simulink model "Raspi_LSTM"  (R2023a)
settings: Solver=FixedStepAuto  StartTime=0.0  StopTime=inf  RelTol=1e-3  EnableMultiTasking=on
InitFcn:
  | timespan=1.5;
  | sampling_subsample=3;
undefined symbols (not defined in the file or in its folder): plughw
libraries: dspvision x8, raspberrypiIOTlib x2, raspberrypiAVlib x1, dspsnks4 x1, deeplib x1, dspfeatures x1
settings Model: SimulationMode=external  ExtModeTrigDuration=2  Creator=tokamoto  LastModifiedBy=tokamoto
settings SolverCC: AlgebraicLoopSolver=TrustRegion  PositivePriorityOrder=on
settings DataIOCC: LimitDataPoints=on  DSMLogging=off  StreamToWks=off  ReturnWorkspaceOutputs=off
settings OptimizationCC: ZeroExternalMemoryAtStartup=off  ZeroInternalMemoryAtStartup=off  MaxStackSize=64
settings DebuggingCC: ParameterTunabilityLossMsg=error  UnconnectedInputMsg=warning  UnconnectedOutputMsg=warning  UnconnectedLineMsg=warning  ArithmeticOperatorsInVariantConditions=warning
settings HardwareCC: ProdBitPerPointer=32  ProdBitPerSizeT=32  ProdBitPerPtrDiffT=32  ProdLargestAtomicInteger=Long  ProdLargestAtomicFloat=Double  ProdWordSize=32  ProdLongLongMode=on  ProdHWDeviceType=ARM Compatible->ARM Cortex
settings ModelReferenceCC: EnableRefExpFcnMdlSchedulingChecks=on
settings SFSimCC: SimUseLocalCustomCode=off  CustomCodeUndefinedFunction=UseInterfaceOnly
settings RTWCC: Description=Embedded Coder  SystemTargetFile=ert.tlc  HardwareBoard=Raspberry Pi  TLCOptions="-aInlineSetEventsForThisBaseRateFcn=TLC_FALSE -aSuppressMultiTaskScheduler=TLC_FALSE  -aRateBasedStepFcn=0"  TemplateMakefile=ert_default_tmf  GenerateReport=on  RTWUseLocalCustomCode=off  Toolchain=GNU GCC Embedded Linux  BuildConfiguration=Faster Runs  LaunchReport=on  GenerateCodeMetricsReport=on
settings CodeAppCC: ForceParamTrailComments=on  OperatorAnnotations=on  StateflowObjectComments=on  MATLABSourceComments=on
settings ERTTargetCC: CodeReplacementLibrary=GCC ARM Cortex-A  ERTCustomFileBanners=off  SupportComplex=off  SupportNonInlinedSFcns=on  RemoveResetFunc=off  SupportVariableSizeSignals=on  ModelStepFunctionPrototypeControlCompliant=off  ExtModeTransport=2  ExtModeStaticAlloc=on  ExtModeMexFile=ext_xcp  ExtModeIntrfLevel=Level2 - Open  RootIOFormat=Structure reference

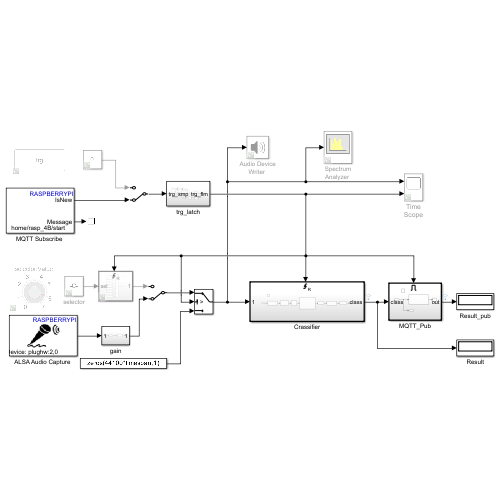
[thumbnail: Simulink's stored preview of the top-level diagram]
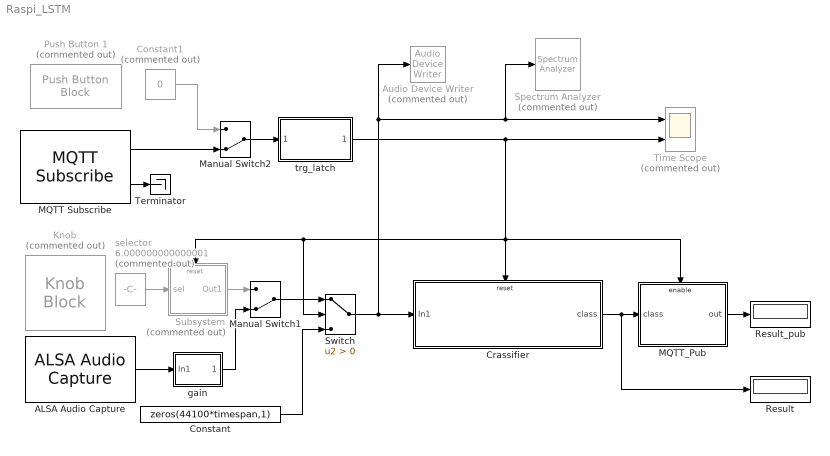
== system Raspi_LSTM ==
  "ALSA Audio Capture " : raspberrypiAVlib/ALSA Audio Capture  deviceStr=plughw:2,0  DataBitDepth=16-bit integer  numberOfChannels=1  sampleRateEnum=44100  frameSize=44100*timespan  QueueDuration=0.5  blockPlatform=LINUX
  "Audio Device Writer " : dspsnks4/Audio Device Writer  Commented=on  Driver=DirectSound  Device=Default  InheritSampleRate=off  SampleRate=44100  BitDepth=16-bit integer  BufferSize=4096  NumBuffers=10  DefaultOutputChannelMapping=on  OutputChannelMapping=1:2  OutputNumUnderrunSamples=off  DriverIdx=1  DeviceWarnFlag=''
  Constant : Constant  Value=zeros(44100*timespan,1)  OutDataTypeStr=single
  Constant1 : Constant  Commented=on  Value=0
  Crassifier : Subsystem  TreatAsAtomicUnit=on
  Knob : KnobBlock  Commented=on  ScaleMax=7  TickInterval=1
  "MQTT Subscribe " : raspberrypiIOTlib/MQTT Subscribe  Topic=home/rasp_4B/start  QoS=0  MessageLength=1  OutputMessage=off  SampleTime=0.5  blockPlatform=RASPBERRYPI
  MQTT_Pub : Subsystem
  Manual Switch1 : ManualSwitch  CurrentSetting=0
  Manual Switch2 : ManualSwitch  CurrentSetting=0
  Push Button 1 : PushButtonBlock  Commented=on  ButtonText=trg  OffValue=0.000000
  Result : Display
  Result_pub : Display
  "Spectrum Analyzer " : SpectrumAnalyzer  Commented=on  WindowPosition=[1101.000000,243.000000,434.000000,391.000000,]  ScopeFrameLocation=window  ViewType=Spectrum and spectrogram  SampleRateSource=Property  SampleRate=44.1e3  PlotAsTwoSidedSpectrum=off  FrequencyScale=Log  FrequencySpan=Start and stop frequencies  StartFrequency=20  StopFrequency=20e3  YLimits=[-181.7430131,-99.5033473]  ColorLimits=[-181.7430131,-99.5033473]  SelectedToolstripTab=spectrumAnalyzerToolstrip.estimationTab  DefaultConfigurationName=spbscopes.SpectrumAnalyzerBlockCfg  IsFrequencyInputMode=0  FrequencyVectorPort=0  FrequencyVectorFromPort=0  FrequencyInputRBWPort=0  FrequencyInputRBWFromPort=0
  Subsystem : Subsystem  Commented=on
  Switch : Switch  Criteria=u2 > Threshold  SaturateOnIntegerOverflow=off  InputSameDT=off
  Terminator : Terminator
  Time Scope : Scope  Commented=on  NumInputPorts=2
  gain : Subsystem
  selector : Constant  Commented=on  Value=6.000000000000001
  trg_latch : Subsystem
  wires:
  "MQTT Subscribe "/2 -> Terminator/1
  Constant1/1 -> Manual Switch2/1
  "MQTT Subscribe "/1 -> Manual Switch2/2
  Manual Switch2/1 -> trg_latch/1(trg_smp)
  Crassifier/1(class) -> MQTT_Pub/1(class), Result/1
  MQTT_Pub/1(out) -> Result_pub/1
  Constant/1 -> Switch/3
  selector/1 -> Subsystem/1(sel)
  Manual Switch1/1 -> Switch/1
  Subsystem/1(Out1) -> Manual Switch1/1
  Switch/1 -> Crassifier/1(In1), "Audio Device Writer "/1, Time Scope/1, "Spectrum Analyzer "/1
  trg_latch/1(trg_flm) -> Time Scope/2, Subsystem/Reset, Switch/2, Crassifier/Reset, MQTT_Pub/Enable
  "ALSA Audio Capture "/1 -> gain/1(In1)
  gain/1(Out1) -> Manual Switch1/2

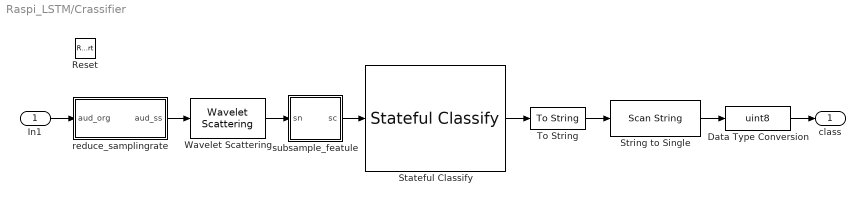
== system Raspi_LSTM/Crassifier ==
  In1 : Inport
  Reset : ResetPort  DisableCoverage=on
  Data Type Conversion : DataTypeConversion  OutDataTypeStr=uint8  SaturateOnIntegerOverflow=off  RndMeth=Floor
  Stateful Classify : deeplib/Stateful Classify  Network=Network from MAT-file  NetworkFunction=untitled  NetworkFilePath=C:\Users\tokamoto\MATLAB\Projects\Raspi\LSTM_Wavelet_MQTT\nefProjectedFinetuned.mat  SampleTime=-1  Classification=on  Predictions=off  ForceInterpretedSim=off  PredictMode=All probabilities and labels  K=5
  String to Single : ScanString  Format="\"x%d_label\""
  To String : ToString
  Wavelet Scattering : dspfeatures/Wavelet Scattering  SignalLength=44100*timespan/sampling_subsample  OverlapLength=0  SpecifySampleRate=on  SampleRate=44100/sampling_subsample  InvarianceScaleSamples=44100/3*0.5  InvarianceScaleSeconds=0.5  QualityFactors=[8,1]  OptimizePath=off  OversamplingFactor=0  Boundary=periodic  IncludeZeroOrderCoeff=off  FeatureMatrixNormalization=none  FeatureMatrixTransform=log
  reduce_samplingrate : MATLAB Function  TreatAsAtomicUnit=on
  subsample_featule : MATLAB Function  TreatAsAtomicUnit=on
  class : Outport
  wires:
  subsample_featule/1(sc) -> Stateful Classify/1
  reduce_samplingrate/1(aud_ss) -> Wavelet Scattering/1
  Data Type Conversion/1 -> class/1
  Wavelet Scattering/1 -> subsample_featule/1(sn)
  String to Single/1 -> Data Type Conversion/1
  Stateful Classify/1 -> To String/1
  To String/1 -> String to Single/1
  In1/1 -> reduce_samplingrate/1(aud_org)

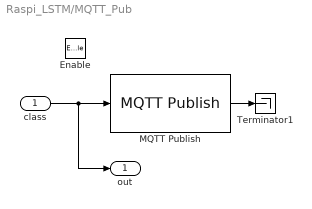
== system Raspi_LSTM/MQTT_Pub ==
  class : Inport
  Enable : EnablePort
  MQTT Publish : raspberrypiIOTlib/MQTT Publish  Topic=home/rasp_4B/state  QoS=0  RetainMsg=on  blockPlatform=RASPBERRYPI
  Terminator1 : Terminator
  out : Outport
  wires:
  MQTT Publish/1 -> Terminator1/1
  class/1 -> out/1, MQTT Publish/1

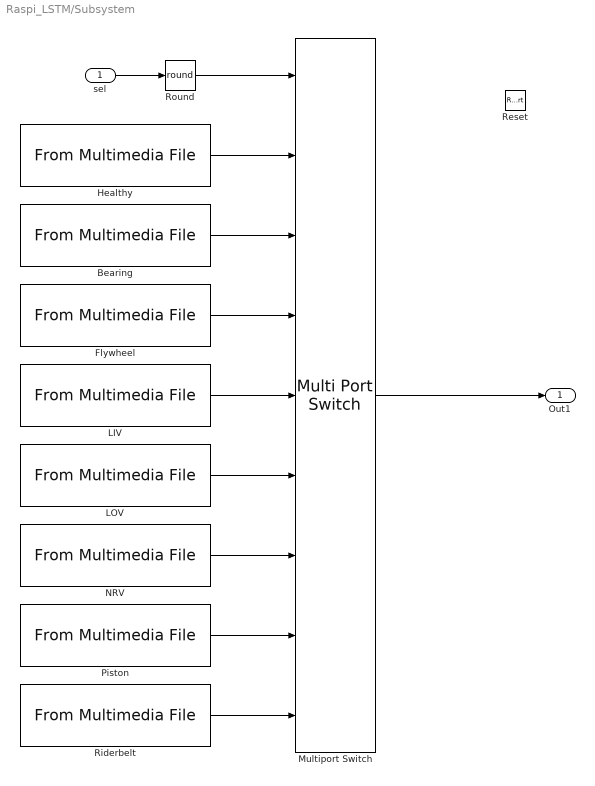
== system Raspi_LSTM/Subsystem ==
  sel : Inport
  Reset : ResetPort  DisableCoverage=on
  Bearing : dspvision/From Multimedia File  inputFilename=1_Bearing.wav  readRange=[1 inf]  loop=on  numPlays=1  outputStreams=オーディオのみ  videoDataType=single  audioDataType=double  inheritSampleTime=on  userDefinedSampleTime=1/16  noAudioOutput=off  isIntensityVideo=off  fourcc=RGB  colorVideoFormat=Separate color signals  outputEOF=off  dataOrg=Column-major  audioFrameSize=44100*timespan  computeAudioFrameSize=off  outSamplingMode=Sample based
  Flywheel : dspvision/From Multimedia File  inputFilename=2_Flywheel.wav  readRange=[1 inf]  loop=on  numPlays=1  outputStreams=オーディオのみ  videoDataType=single  audioDataType=double  inheritSampleTime=on  userDefinedSampleTime=1/16  noAudioOutput=off  isIntensityVideo=off  fourcc=RGB  colorVideoFormat=Separate color signals  outputEOF=off  dataOrg=Column-major  audioFrameSize=44100*timespan  computeAudioFrameSize=off  outSamplingMode=Sample based
  Healthy : dspvision/From Multimedia File  inputFilename=0_Healthy.wav  readRange=[1 inf]  loop=on  numPlays=1  outputStreams=オーディオのみ  videoDataType=single  audioDataType=double  inheritSampleTime=on  userDefinedSampleTime=1/16  noAudioOutput=off  isIntensityVideo=off  fourcc=RGB  colorVideoFormat=Separate color signals  outputEOF=off  dataOrg=Column-major  audioFrameSize=44100*timespan  computeAudioFrameSize=off  outSamplingMode=Sample based
  LIV : dspvision/From Multimedia File  inputFilename=3_LIV.wav  readRange=[1 inf]  loop=on  numPlays=1  outputStreams=オーディオのみ  videoDataType=single  audioDataType=double  inheritSampleTime=on  userDefinedSampleTime=1/16  noAudioOutput=off  isIntensityVideo=off  fourcc=RGB  colorVideoFormat=Separate color signals  outputEOF=off  dataOrg=Column-major  audioFrameSize=44100*timespan  computeAudioFrameSize=off  outSamplingMode=Sample based
  LOV : dspvision/From Multimedia File  inputFilename=4_LOV.wav  readRange=[1 inf]  loop=on  numPlays=1  outputStreams=オーディオのみ  videoDataType=single  audioDataType=double  inheritSampleTime=on  userDefinedSampleTime=1/16  noAudioOutput=off  isIntensityVideo=off  fourcc=RGB  colorVideoFormat=Separate color signals  outputEOF=off  dataOrg=Column-major  audioFrameSize=44100*timespan  computeAudioFrameSize=off  outSamplingMode=Sample based
  Multiport Switch : MultiPortSwitch  DataPortOrder=Zero-based contiguous  Inputs=8  DiagnosticForDefault=None  zeroidx=on  SaturateOnIntegerOverflow=off  InputSameDT=off
  NRV : dspvision/From Multimedia File  inputFilename=5_NRV.wav  readRange=[1 inf]  loop=on  numPlays=1  outputStreams=オーディオのみ  videoDataType=single  audioDataType=double  inheritSampleTime=on  userDefinedSampleTime=1/16  noAudioOutput=off  isIntensityVideo=off  fourcc=RGB  colorVideoFormat=Separate color signals  outputEOF=off  dataOrg=Column-major  audioFrameSize=44100*timespan  computeAudioFrameSize=off  outSamplingMode=Sample based
  Piston : dspvision/From Multimedia File  inputFilename=6_Piston.wav  readRange=[1 inf]  loop=on  numPlays=1  outputStreams=オーディオのみ  videoDataType=single  audioDataType=double  inheritSampleTime=on  userDefinedSampleTime=1/16  noAudioOutput=off  isIntensityVideo=off  fourcc=RGB  colorVideoFormat=Separate color signals  outputEOF=off  dataOrg=Column-major  audioFrameSize=44100*timespan  computeAudioFrameSize=off  outSamplingMode=Sample based
  Riderbelt : dspvision/From Multimedia File  inputFilename=7_Riderbelt.wav  readRange=[1 inf]  loop=on  numPlays=1  outputStreams=オーディオのみ  videoDataType=single  audioDataType=double  inheritSampleTime=on  userDefinedSampleTime=1/16  noAudioOutput=off  isIntensityVideo=off  fourcc=RGB  colorVideoFormat=Separate color signals  outputEOF=off  dataOrg=Column-major  audioFrameSize=44100*timespan  computeAudioFrameSize=off  outSamplingMode=Sample based
  Round : Rounding  Operator=round
  Out1 : Outport
  wires:
  sel/1 -> Round/1
  LOV/1 -> Multiport Switch/6
  NRV/1 -> Multiport Switch/7
  Healthy/1 -> Multiport Switch/2
  LIV/1 -> Multiport Switch/5
  Bearing/1 -> Multiport Switch/3
  Flywheel/1 -> Multiport Switch/4
  Round/1 -> Multiport Switch/1
  Riderbelt/1 -> Multiport Switch/9
  Piston/1 -> Multiport Switch/8
  Multiport Switch/1 -> Out1/1

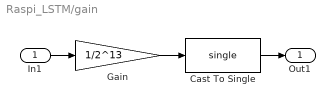
== system Raspi_LSTM/gain ==
  In1 : Inport
  Cast To Single : DataTypeConversion  OutDataTypeStr=single  SaturateOnIntegerOverflow=off  RndMeth=Floor
  Gain : Gain  Gain=1/2^13
  Out1 : Outport
  wires:
  Cast To Single/1 -> Out1/1
  Gain/1 -> Cast To Single/1
  In1/1 -> Gain/1

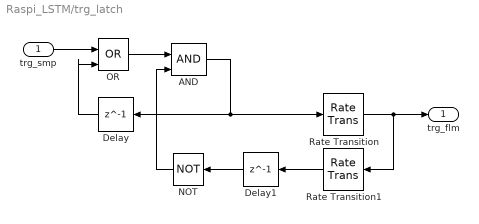
== system Raspi_LSTM/trg_latch ==
  trg_smp : Inport
  AND : Logic  IconShape=distinctive  AllPortsSameDT=off  OutDataTypeStr=boolean
  Delay : Delay  DelayLength=1
  Delay1 : Delay  DelayLength=1
  NOT : Logic  Operator=NOT  IconShape=distinctive  AllPortsSameDT=off  OutDataTypeStr=boolean
  OR : Logic  Operator=OR  IconShape=distinctive  AllPortsSameDT=off  OutDataTypeStr=boolean
  Rate Transition : RateTransition  Deterministic=off  OutPortSampleTimeOpt=Inherit
  Rate Transition1 : RateTransition  Deterministic=off  OutPortSampleTimeOpt=Inherit
  trg_flm : Outport
  wires:
  AND/1 -> Delay/1, Rate Transition/1
  Rate Transition/1 -> trg_flm/1, Rate Transition1/1
  OR/1 -> AND/1
  Rate Transition1/1 -> Delay1/1
  NOT/1 -> AND/2
  Delay/1 -> OR/2
  trg_smp/1 -> OR/1
  Delay1/1 -> NOT/1

== matlab function Raspi_LSTM/Crassifier/reduce_samplingrate ==
  data: aud_org input; aud_ss output
function aud_ss = fcn(aud_org)
sampling_subsample=3; % 44100Hz-> 14700Hz
aud_ss = single(aud_org(1:sampling_subsample:end,:));

== matlab function Raspi_LSTM/Crassifier/subsample_featule ==
  data: sn input; sc output
function sc = fcn(sn)
feature_subsample=2;
sc = sn(:,1:feature_subsample:end);
